simulink model "EV_thermal_charger_2015a_20200311"  (R2015a)
settings: Solver=ode3  StartTime=0.0  StopTime=1800  FixedStep=sampling_time  RelTol=1e-3
PreLoadFcn:
  | run('init_setting.m')
PostLoadFcn:
  | set_param(gcs, 'SimulationCommand', 'update');
  | load('save_param/save_P_Charger', 'P_Charger');
  | load('save_param/save_T_User_set_temp_degC','T_User_set_temp_degC');
  | load('save_param/save_ENV_PNT_PTTH_Temp_add_degC','ENV_PNT_PTTH_Temp_add_degC');
  | load('save_param/save_ENV_PNT_CABIN_Temp_add_degC','ENV_PNT_CABIN_Temp_add_degC');
  | load('save_param/save_ENV_PNT_PHI_Sunlight_W','ENV_PNT_PHI_Sunlight_W');
  | load('save_param/save_ENV_PNT_Outside_Temp_ini_degC','ENV_PNT_Outside_Temp_ini_degC');
undefined symbols (not defined in the file or in its folder): BK_PNT_Pow_UL, BK_PNT_ReGene_vel_limit_DN_kmph, BK_PNT_ReGene_vel_limit_UP_kmph, BK_PNT_Tau_brake, Brk_LL, Brk_PGain, Brk_UL, BT_PNT_Hi_C_pol_hi_batt, BT_PNT_Hi_Capa_hi_batt_F, BT_PNT_Hi_ocv_SOC_hi_batt_OCV_V_table, BT_PNT_Hi_ocv_SOC_hi_batt_OCV_V_table_x_SOC, BT_PNT_Hi_R_hi_batt_cell, BT_PNT_Hi_R_pol_hi_batt, BT_PNT_Hi_SOC_MAX_hi_batt, BT_PNT_Hi_SOC_MIN_hi_batt, BT_PNT_Hi_SOC_START_hi_batt, BT_PNT_Lo_Capa_lo_batt_F, BT_PNT_Lo_ocv_SOC_lo_batt_OCV_V_table, BT_PNT_Lo_ocv_SOC_lo_batt_OCV_V_table_x_SOC, BT_PNT_Lo_R_lo_batt_ohm, BT_PNT_Lo_SOC_MAX_lo_batt, BT_PNT_Lo_SOC_MIN_lo_batt, BT_PNT_Lo_SOC_START_lo_batt, BTTH_CNT_P_BT_Heater_W, BTTH_CNT_P_BT_Heater_W_x_BTCells_degC, BTTH_CNT_Voltage_BTFan_V, BTTH_CNT_Voltage_BTFan_V_x_BTCells_degC, BTTH_PNT_BT_Heat_Resi_KpW, BTTH_PNT_BT_Heat_Resi_KpW_x_Wind_m3ps, BTTH_PNT_BT_Heater2BTCells_Heat_Resi_KpW, BTTH_PNT_BT_Heater_Heat_Capa_JpK, BTTH_PNT_BTBlock2BTAir_Heat_Resi_KpW, BTTH_PNT_BTBlock_Heat_Capa_JpK, BTTH_PNT_BTCells2BTBlock_Heat_Resi_KpW, BTTH_PNT_BTCells_Heat_Capa_JpK, BTTH_PNT_v_BTFan_Wind_vel_mps, BTTH_PNT_v_BTFan_Wind_vel_mps_x_V_BTFan, CATH_CNT_P_Aircon_W_LL, CATH_CNT_P_Aircon_W_UL, CATH_CNT_P_Gain_Aircon, CATH_CNT_P_Gain_PTC_Heater, CATH_CNT_P_Gain_SeatHT, CATH_CNT_P_PTC_Heater, CATH_CNT_P_PTC_Heater_W_LL, CATH_CNT_P_PTC_Heater_W_UL, CATH_CNT_P_PTC_Heater_x_T_Outside_temp_degC, CATH_CNT_P_SeatHT_W_LL, CATH_CNT_P_SeatHT_W_UL, CATH_CNT_PGain_Temp_blowout, CATH_CNT_T_Aircon_Indoor_degC, CATH_CNT_T_Aircon_Indoor_degC_x_T_blowout_degC, CATH_CNT_T_PTC_Heater_degC_UL, CATH_CNT_T_SeatHT_Temp_degC, CATH_CNT_T_SeatHT_Temp_degC_x_T_blowout_degC, CATH_CNT_V_HVAC_Fan, CATH_CNT_V_HVAC_Fan_x_T_blowout_degC, CATH_CNT_V_RDFan_V, CATH_CNT_V_RDFan_x_P_Aircon_W, CATH_PNT_Air_Convection_Heat_Resi_KpW, CATH_PNT_Air_Convection_Heat_Resi_x_mps ... (+141)
undefined symbols (not defined in the file): ACC_D_Gain, ACC_I_Gain, ACC_P_Gain
libraries: METI_Lib_vehicle_model x52, simulink x35
(part 1 of 6)
PreSaveFcn:
  | save('save_param/save_P_Charger', 'P_Charger');
  | save('save_param/save_T_User_set_temp_degC', 'T_User_set_temp_degC');
  | save('save_param/save_ENV_PNT_PTTH_Temp_add_degC', 'ENV_PNT_PTTH_Temp_add_degC');
  | save('save_param/save_ENV_PNT_CABIN_Temp_add_degC', 'ENV_PNT_CABIN_Temp_add_degC');
  | save('save_param/save_ENV_PNT_PHI_Sunlight_W', 'ENV_PNT_PHI_Sunlight_W');
  | save('save_param/save_ENV_PNT_Outside_Temp_ini_degC', 'ENV_PNT_Outside_Temp_ini_degC');
settings Model: Creator=AZAPA  LastModifiedBy=itc-38
settings OptimizationCC: EfficientMapNaN2IntZero=off
settings DebuggingCC: SFInvalidInputDataAccessInChartInitDiag=none  SFNoUnconditionalDefaultTransitionDiag=none
settings HardwareCC: TargetLongLongMode=on  TargetIntDivRoundTo=Zero  TargetEndianess=LittleEndian  TargetHWDeviceType=MATLAB Host  ProdEqTarget=off
settings CodeAppCC: MaxIdLength=128
settings GRTTargetCC: CombineOutputUpdateFcns=off  GRTInterface=on

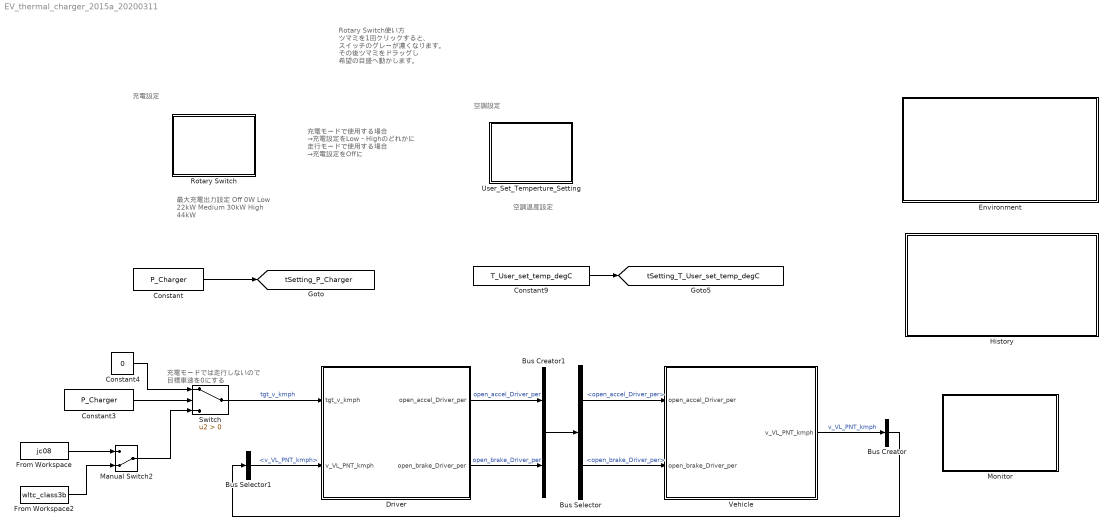
== system EV_thermal_charger_2015a_20200311 ==
  note: 充電モードでは走行しないので
      | 目標車速を0にする
  note: 充電モードで使用する場合
      | →充電設定をLow～Highのどれかに
      |
      | 走行モードで使用する場合
      | →充電設定をOffに
  note: 充電設定
  note: 空調温度設定
  note: 空調設定
  note: 最大充電出力設定
      | Off 0W
      | Low 22kW
      | Medium 30kW
      | High 44kW
  note: Rotary Switch使い方
      | ツマミを1回クリックすると、
      | スイッチのグレーが濃くなります。
      | その後ツマミをドラッグし
      | 希望の目盛へ動かします。
  Bus Creator : BusCreator  Inputs=1
  Bus Creator1 : BusCreator  Inputs=2
  Bus Selector : BusSelector  OutputSignals=open_accel_Driver_per,open_brake_Driver_per
  Bus Selector1 : BusSelector  OutputSignals=v_VL_PNT_kmph
  Constant : Constant  Value=P_Charger
  Constant3 : Constant  Value=P_Charger
  Constant4 : Constant  Value=0
  Constant9 : Constant  Value=T_User_set_temp_degC
  Driver : Subsystem
      mask Display: image(imread('picture\ドライバ.png'))
  Environment : Subsystem
  From Workspace : FromWorkspace  VariableName=jc08  SampleTime=0
  From Workspace2 : FromWorkspace  VariableName=wltc_class3b  SampleTime=0
  History : Subsystem
  Manual Switch2 : ManualSwitch  CurrentSetting=0
  Monitor : Subsystem
  Rotary Switch : Subsystem  DialogController=hmiCreateDDGDialog  IsWebBlock=on  mask(MathWorksWebBlock){webBlockId=86bdfb7e-e008-490f-bc47-d07dc2166084, webBlockType=discreteknob, ShowInLibBrowser=on, ShowInitialText=on, HMISrcModelName=EV_thermal_charger_2015a_20200311}
      mask prompts: webBlockId "WebBlock Id"; webBlockType "WebBlock Type"; HMISrcModelName "Source Model"
      mask Help: helpview([docroot '/mapfiles/simulink.map'], 'hmi_rotary_switch')
      mask Display:
      | model = bdroot(gcb);
      | if strcmp(get_param(model,'BlockDiagramType'), 'library')
      |     image([(matlabroot) '/toolbox/simulink/hmi/icons/DiscreteKnob.png']);
      | end
  Switch : Switch  Criteria=u2 > Threshold
  User_Set_Temperture_Setting : Subsystem  DialogController=hmiCreateDDGDialog  IsWebBlock=on  mask(MathWorksWebBlock){webBlockId=2ed6c567-8d1a-4bfe-bbc2-8860f67c8545, webBlockType=discreteknob, ShowInLibBrowser=on, ShowInitialText=on, HMISrcModelName=EV_thermal_charger_2015a_20200311}
      mask prompts: webBlockId "WebBlock Id"; webBlockType "WebBlock Type"; HMISrcModelName "Source Model"
      mask help: 値を設定してパラメーターまたは変数を調整します。
      mask Help: helpview([docroot '/mapfiles/simulink.map'], 'hmi_rotary_switch')
      mask Display:
      | if strcmp(get_param(bdroot(gcb),'BlockDiagramType'),'library')
      |  image([(matlabroot) '/toolbox/simulink/hmi/icons/DiscreteKnob.png'])
      | end
  Vehicle : Subsystem
      mask Display: image(imread('picture\電気負荷.png'))
  tag scope: tSetting_P_Charger=global, tSetting_T_User_set_temp_degC=global
  wires:
  Switch/1 -> Driver/1(tgt_v_kmph)  "tgt_v_kmph"
  From Workspace/1 -> Manual Switch2/1
  From Workspace2/1 -> Manual Switch2/2
  Vehicle/1(v_VL_PNT_kmph) -> Bus Creator/1  "v_VL_PNT_kmph"
  Bus Selector/1 -> Vehicle/1(open_accel_Driver_per)  "<open_accel_Driver_per>"
  Bus Selector/2 -> Vehicle/2(open_brake_Driver_per)  "<open_brake_Driver_per>"
  Bus Creator1/1 -> Bus Selector/1
  Driver/1(open_accel_Driver_per) -> Bus Creator1/1  "open_accel_Driver_per"
  Driver/2(open_brake_Driver_per) -> Bus Creator1/2  "open_brake_Driver_per"
  Bus Creator/1 -> Bus Selector1/1
  Bus Selector1/1 -> Driver/2(v_VL_PNT_kmph)  "<v_VL_PNT_kmph>"
  Manual Switch2/1 -> Switch/3
  Constant3/1 -> Switch/2
  Constant4/1 -> Switch/1
  Constant/1 -> [tSetting_P_Charger]
  Constant9/1 -> [tSetting_T_User_set_temp_degC]

== system EV_thermal_charger_2015a_20200311/Driver ==
  tgt_v_kmph : Inport
  v_VL_PNT_kmph : Inport  Port=2
  Caliculate_Driving_State : Subsystem
  Caliculate_Opeining_Accel : Subsystem
  Caliculate_Opening_Brake : Subsystem
  Memory2 : Memory  InheritSampleTime=on
  open_accel_Driver_per : Outport
  open_brake_Driver_per : Outport  Port=2
  tag scope: tScope_accel=global, tScope_brake=global, tScope_v_Vehicle=global, tScope_v_tgt=global
  wires:
  tgt_v_kmph/1 -> Caliculate_Driving_State/2(tgt_v_kmph), Caliculate_Opening_Brake/2(tgt_v_kmph), Caliculate_Opeining_Accel/2(tgt_v_kmph), [tScope_v_tgt]
  Memory2/1 -> [tScope_v_Vehicle], Caliculate_Opening_Brake/1(v_VL_PNT_kmph), Caliculate_Opeining_Accel/1(v_VL_PNT_kmph)
  Caliculate_Opeining_Accel/1(open_accel_Driver_per) -> open_accel_Driver_per/1, [tScope_accel], Caliculate_Opening_Brake/3(open_accel_Driver_per)
  Caliculate_Opening_Brake/1(open_brake_Driver_per) -> open_brake_Driver_per/1, [tScope_brake], Caliculate_Driving_State/1(open_brake_Driver_per)
  v_VL_PNT_kmph/1 -> Memory2/1

== system EV_thermal_charger_2015a_20200311/Environment ==
  note: 車外気温設定
      | VeryCold -30℃
      | Cold 0℃
      | Warm 20℃
      | VeryHot 40℃
  note: 気象設定（直射日光の有無）
      | Night 日射熱量 0W
      | Cloudy 日射熱量 100W
      | Sunny 日射熱量 1000W
  note: 気象条件設定
  note: Rotary Switch使い方
      | ツマミを1回クリックすると、
      | スイッチのグレーが濃くなります。
      | その後ツマミをドラッグし
      | 希望の目盛へ動かします。
  note: スタート時
      | 車室温度設定
      | 直射日光下で駐車した状態では
      | 車室温度は外気温より高くなる
  note: スタート時パワトレ・パワエレ
      | HOT/COLD設定
      | COLD 外気温と同じ温度から
      | HOT 外気温+40℃から
  note: 車両条件設定
  CABIN_Temp_add : Subsystem  DialogController=hmiCreateDDGDialog  IsWebBlock=on  mask(MathWorksWebBlock){webBlockId=d78e8cf1-5ca2-40c7-aa2c-f2b450f5124d, webBlockType=discreteknob, ShowInLibBrowser=on, ShowInitialText=on, HMISrcModelName=[]}
      mask prompts: webBlockId "WebBlock Id"; webBlockType "WebBlock Type"; HMISrcModelName "Source Model"
      mask help: 値を設定してパラメーターまたは変数を調整します。
      mask Help: helpview([docroot '/mapfiles/simulink.map'], 'hmi_rotary_switch')
      mask Display:
      | if strcmp(get_param(bdroot(gcb),'BlockDiagramType'),'library')
      |  image([(matlabroot) '/toolbox/simulink/hmi/icons/DiscreteKnob.png'])
      | end
  COLD/HOT : Subsystem  DialogController=hmiCreateDDGDialog  IsWebBlock=on  mask(MathWorksWebBlock){webBlockId=64b15bba-436a-47d2-9f2c-332ccf488184, webBlockType=discreteknob, ShowInLibBrowser=on, ShowInitialText=on, HMISrcModelName=[]}
      mask prompts: webBlockId "WebBlock Id"; webBlockType "WebBlock Type"; HMISrcModelName "Source Model"
      mask help: 値を設定してパラメーターまたは変数を調整します。
      mask Help: helpview([docroot '/mapfiles/simulink.map'], 'hmi_rotary_switch')
      mask Display:
      | if strcmp(get_param(bdroot(gcb),'BlockDiagramType'),'library')
      |  image([(matlabroot) '/toolbox/simulink/hmi/icons/DiscreteKnob.png'])
      | end
  Constant5 : Constant  Value=ENV_PNT_PTTH_Temp_add_degC
  Constant6 : Constant  Value=ENV_PNT_CABIN_Temp_add_degC
  Constant7 : Constant  Value=ENV_PNT_PHI_Sunlight_W
  Constant8 : Constant  Value=ENV_PNT_Outside_Temp_ini_degC
  Outside_Temperture_Setting : Subsystem  DialogController=hmiCreateDDGDialog  IsWebBlock=on  mask(MathWorksWebBlock){webBlockId=e3e71119-3dae-4264-804d-d3a93d53d578, webBlockType=discreteknob, ShowInLibBrowser=on, ShowInitialText=on, HMISrcModelName=[]}
      mask prompts: webBlockId "WebBlock Id"; webBlockType "WebBlock Type"; HMISrcModelName "Source Model"
      mask help: 値を設定してパラメーターまたは変数を調整します。
      mask Help: helpview([docroot '/mapfiles/simulink.map'], 'hmi_rotary_switch')
      mask Display:
      | if strcmp(get_param(bdroot(gcb),'BlockDiagramType'),'library')
      |  image([(matlabroot) '/toolbox/simulink/hmi/icons/DiscreteKnob.png'])
      | end
  Sunlight_Heat_Flux_Setting : Subsystem  DialogController=hmiCreateDDGDialog  IsWebBlock=on  mask(MathWorksWebBlock){webBlockId=802d8e5a-7805-4abc-9448-1c2511a8212f, webBlockType=discreteknob, ShowInLibBrowser=on, ShowInitialText=on, HMISrcModelName=[]}
      mask prompts: webBlockId "WebBlock Id"; webBlockType "WebBlock Type"; HMISrcModelName "Source Model"
      mask help: 値を設定してパラメーターまたは変数を調整します。
      mask Help: helpview([docroot '/mapfiles/simulink.map'], 'hmi_rotary_switch')
      mask Display:
      | if strcmp(get_param(bdroot(gcb),'BlockDiagramType'),'library')
      |  image([(matlabroot) '/toolbox/simulink/hmi/icons/DiscreteKnob.png'])
      | end
  tag scope: PHI_Environment_Sunlight_W=global, add_T_Environment_CATH_degC=global, add_T_Environment_PTTH_ELTH_degC=global, ini_T_Environment_Outside_degC=global
  wires:
  Constant7/1 -> [PHI_Environment_Sunlight_W]
  Constant8/1 -> [ini_T_Environment_Outside_degC]
  Constant5/1 -> [add_T_Environment_PTTH_ELTH_degC]
  Constant6/1 -> [add_T_Environment_CATH_degC]

== system EV_thermal_charger_2015a_20200311/History ==

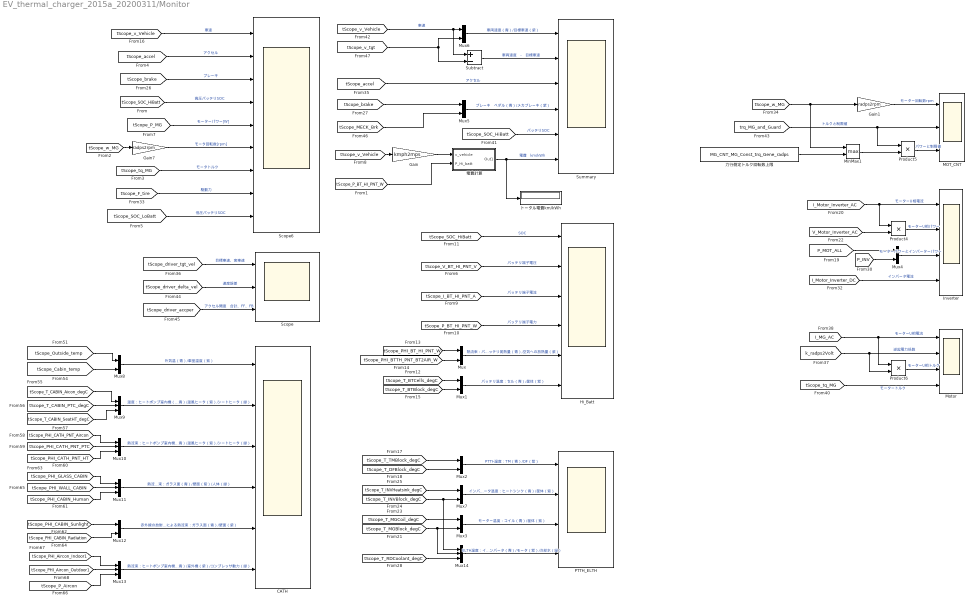
== system EV_thermal_charger_2015a_20200311/Monitor ==
  CATH : Scope  NumInputPorts=6
      settings: YMin=20~20~-35000~-0~0~-15000  YMax=70~70~5000~4500~1000~35000  SaveName=ScopeData12
  Gain : Gain  Gain=kmph2mps
  Gain1 : Gain  Gain=radps2rpm
  Gain7 : Gain  Gain=radps2rpm
  Hi_Batt : Scope  NumInputPorts=6
      settings: YMin=44.5~337.5~-100~-40000~-100~20  YMax=50~352.5~125~40000~1000~20.4  SaveName=ScopeData4
  Inverter : Scope  NumInputPorts=4
      settings: TimeRange=1800  YMin=-30~-7500~-12500~-30  YMax=60~15000~22500~60  SaveName=ScopeData15
  MOT_CNT : Scope  NumInputPorts=3
      settings: TimeRange=1800  YMin=-500~-350~-125000  YMax=7000~350~125000  SaveName=ScopeData11
  MinMax1 : MinMax  Function=max  Inputs=2
  Motor : Scope  NumInputPorts=4
      settings: TimeRange=1800  YMin=-2.5~0.75~-5~-10  YMax=35~1.025~40~100  SaveName=ScopeData14
  Mux{,1..8,12} (10 alike) : Mux  Inputs=2
  Mux{9..11,13..14} (5 alike) : Mux  Inputs=3
  PTTH_ELTH : Scope  NumInputPorts=4
      settings: TimeRange=1800  YMin=40~40~40~40  YMax=41~41.75~42~42  SaveName=ScopeData10
  Product4 : Product
  Product5 : Product
  Product6 : Product
  Scope : Scope  NumInputPorts=3
      settings: TimeRange=1800  YMin=0~-0.4~-20  YMax=140~1.2~80  SaveName=ScopeData8
  Scope6 : Scope  NumInputPorts=9
      settings: TimeRange=186.7025  YMin=35~0~-1~45.37~-30000~2250~-100~-3000~74.175  YMax=55~50~1~45.48~30000~4000~100~2000~74.35  SaveName=ScopeData6
  Subtract : Sum  Inputs=+-
  Summary : Scope  NumInputPorts=6
      settings: YMin=0~-0.6~0~0~41~0  YMax=150~0.1~70~5~50~9  SaveName=ScopeData5
  トータル電費km/kWh : Display
  力行側定トルク回転数上限 : Constant  Value=MG_CNT_MG_Const_trq_Gene_radps
  電費計算 : Subsystem
  wires:
  [tScope_v_Vehicle] -> Scope6/1  "車速"
  [tScope_accel] -> Scope6/2  "アクセル"
  [tScope_brake] -> Scope6/3  "ブレーキ"
  [tScope_SOC_HiBatt] -> Scope6/4  "高圧バッテリSOC"
  Gain7/1 -> Scope6/6  "モータ回転数[rpm]"
  [tScope_tq_MG] -> Scope6/7  "モータトルク"
  [tScope_F_tire] -> Scope6/8  "駆動力"
  Mux4/1 -> Inverter/3  "モーターパワーとインバーターパワー"
  [I_Motor_Inverter_AC] -> Product4/1, Inverter/1  "モーターU相電流"
  Product4/1 -> Inverter/2  "モーターU相パワー"
  [V_Motor_Inverter_AC] -> Product4/2
  [P_MOT_ALL] -> Mux4/1
  [P_INV] -> Mux4/2
  [I_Motor_Inverter_DC] -> Inverter/4  "インバータ電流"
  [trq_MG_and_Guard] -> Product5/1, MOT_CNT/2  "トルクと制限値"
  Product5/1 -> MOT_CNT/3  "パワーと制限値"
  力行側定トルク回転数上限/1 -> MinMax1/2
  MinMax1/1 -> Product5/2
  Gain1/1 -> MOT_CNT/1  "モーター回転数rpm"
  [tScope_w_MG] -> MinMax1/1, Gain1/1
  [I_MG_AC] -> Product6/1, Motor/1  "モーターU相電流"
  [k_radps2Volt] -> Product6/2, Motor/2  "逆起電力係数"
  Product6/1 -> Motor/3  "モーターU相トルク"
  [tScope_tq_MG] -> Motor/4  "モータートルク"
  Mux5/1 -> Summary/4  "ブレーキ　ペダル（青）/メカブレーキ（紫）"
  [tScope_MECK_Brk] -> Mux5/2
  [tScope_v_Vehicle] -> Subtract/1, Mux6/1  "車速"
  Mux6/1 -> Summary/1  "車両速度（青）/目標車速（紫）"
  Subtract/1 -> Summary/2  "車両速度　-　目標車速"
  [tScope_SOC_HiBatt] -> Summary/5  "バッテリSOC"
  [tScope_v_tgt] -> Mux6/2, Subtract/2
  [tScope_accel] -> Summary/3  "アクセル"
  [tScope_brake] -> Mux5/1
  [tScope_w_MG] -> Gain7/1
  [tScope_driver_tgt_vel] -> Scope/1  "目標車速、実車速"
  [tScope_driver_delta_vel] -> Scope/2  "速度誤差"
  [tScope_driver_accper] -> Scope/3  "アクセル開度　合計、FF、FB"
  電費計算/1(Out1) -> トータル電費km/kWh/1, Summary/6  "電費　km/kWh"
  [tScope_Outside_temp] -> Mux8/1
  [tScope_Cabin_temp] -> Mux8/2
  Mux8/1 -> CATH/1  "外気温（青）/車室温度（紫）"
  Mux9/1 -> CATH/2  "温度：ヒートポンプ室内機（青）/温風ヒータ（紫）/シートヒータ（緑）"
  [tScope_T_CABIN_Aicon_degC] -> Mux9/1
  [tScope_T_CABIN_PTC_degC] -> Mux9/2
  [tScope_T_CABIN_SeatHT_degC] -> Mux9/3
  Mux10/1 -> CATH/3  "熱流束：ヒートポンプ室内機（青）/温風ヒータ（紫）/シートヒータ（緑）"
  [tScope_PHI_CATH_PNT_Aircon] -> Mux10/1
  [tScope_PHI_CATH_PNT_PTC] -> Mux10/2
  [tScope_PHI_CATH_PNT_HT] -> Mux10/3
  Mux11/1 -> CATH/4  "熱流束：ガラス面（青）/壁面（紫）/人体（緑）"
  Mux12/1 -> CATH/5  "赤外線の放射による熱流束：ガラス面（青）/壁面（紫）"
  [tScope_PHI_CABIN_Sunlight] -> Mux12/1
  [tScope_PHI_CABIN_Radiation] -> Mux12/2
  [tScope_PHI_WALL_CABIN] -> Mux11/2
  [tScope_PHI_GLASS_CABIN] -> Mux11/1
  [tScope_PHI_CABIN_Human] -> Mux11/3
  Mux13/1 -> CATH/6  "熱流束：ヒートポンプ室内機（青）/室外機（紫）/コンプレッサ動力（緑）"
  [tScope_PHI_Aircon_Outdoor1] -> Mux13/2
  [tScope_PHI_Aircon_Indoor1] -> Mux13/1
  [tScope_P_Aircon] -> Mux13/3
  [tScope_v_Vehicle] -> Gain/1
  [tScope_P_BT_HI_PNT_W] -> 電費計算/2(P_Hi_batt)
  [tScope_SOC_LoBatt] -> Scope6/9  "低圧バッテリSOC"
  [tScope_P_MG] -> Scope6/5  "モーターパワー[W]"
  [tScope_SOC_HiBatt] -> Hi_Batt/1  "SOC"
  [tScope_V_BT_HI_PNT_V] -> Hi_Batt/2  "バッテリ端子電圧"
  [tScope_I_BT_HI_PNT_A] -> Hi_Batt/3  "バッテリ端子電流"
  Mux1/1 -> Hi_Batt/6  "バッテリ温度：セル（青）/筐体（紫）"
  Mux/1 -> Hi_Batt/5  "熱流束：バッテリ発熱量（青）/空気への放熱量（紫）"
  [tScope_P_BT_HI_PNT_W] -> Hi_Batt/4  "バッテリ端子電力"
  [tScope_PHI_BT_HI_PNT_W] -> Mux/1
  [tScope_PHI_BTTH_PNT_BT2AIR_W] -> Mux/2
  [tScope_T_BTCells_degC] -> Mux1/1
  [tScope_T_BTBlock_degC] -> Mux1/2
  Gain/1 -> 電費計算/1(v_vehicle)
  [tScope_T_DFBlock_degC] -> Mux2/2
  [tScope_T_TMBlock_degC] -> Mux2/1
  [tScope_T_MGCoil_degC] -> Mux3/1
  [tScope_T_MGBlock_degC] -> Mux14/2, Mux3/2
  [tScope_T_INVHeatsink_degC] -> Mux7/1
  [tScope_T_INVBlock_degC] -> Mux14/1, Mux7/2
  [tScope_T_RDCoolant_degC] -> Mux14/3
  Mux2/1 -> PTTH_ELTH/1  "PTTH温度：TM（青）/DF（紫）"
  Mux7/1 -> PTTH_ELTH/2  "インバータ温度：ヒートシンク（青）/筐体（紫）"
  Mux3/1 -> PTTH_ELTH/3  "モーター温度：コイル（青）/筐体（紫）"
  Mux14/1 -> PTTH_ELTH/4  "ELTH温度：インバータ（青）/モータ（紫）/冷却水（緑）"

== system EV_thermal_charger_2015a_20200311/Rotary Switch ==

== system EV_thermal_charger_2015a_20200311/User_Set_Temperture_Setting ==

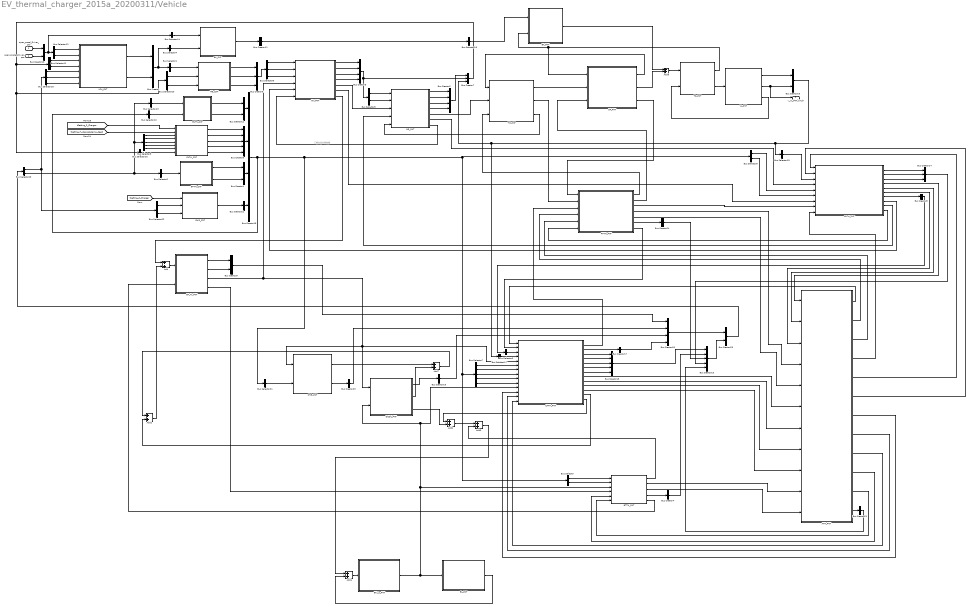
== system EV_thermal_charger_2015a_20200311/Vehicle ==
  note: 三相交流の実効値
  open_accel_Driver_per : Inport
  open_brake_Driver_per : Inport  Port=2
  ATM_PNT : Subsystem
  Add{,1..5,7} (7 alike) : Sum
  BK_CNT : Subsystem
      mask Display: image(imread('picture\ECU02.png'))
  BK_PNT : Subsystem
      mask Display: image(imread('picture\ブレーキ02.png'))
  BTTH_CNT : Subsystem
      mask Display: image(imread('ECU.png'))
  BTTH_PNT : Subsystem
      mask Display: image(imread('Li-INOバッテリ.png'))
  BT_Hi_PNT : Subsystem
      mask Display: image(imread('Li-INOバッテリ.png'))
  BT_Lo_PNT : Subsystem
      mask Display: image(imread('picture\バッテリー.png'))
  Bus Creator{,1,9..10,12,16,25} (7 alike) : BusCreator  Inputs=2
  Bus Creator{4,8,11,17,19,21..24} (9 alike) : BusCreator  Inputs=1
  Bus Creator13 : BusCreator  Inputs=5
  Bus Creator14 : BusCreator  Inputs=3
  Bus Creator15 : BusCreator  Inputs=5
  Bus Creator{2..3,18,20} (4 alike) : BusCreator
  Bus Creator5 : BusCreator  Inputs=5
  Bus Creator6 : BusCreator  Inputs=3
  Bus Creator7 : BusCreator  Inputs=3
  Bus Selector : BusSelector  OutputSignals=signal3.tgt_P_BTTH_CNT_BTHeater_W,signal3.V_BTTH_CNT_BTFan_V
  Bus Selector1 : BusSelector  OutputSignals=tgt_Trq_VCU_CNT_MG_Nm
  Bus Selector10 : BusSelector  OutputSignals=signal2.req_V_CATH_CNT_RDFan_V
  Bus Selector11 : BusSelector  OutputSignals=signal3.v_VL_PNT_mps_1,signal1.w_MG_PNT_radps
  Bus Selector12 : BusSelector  OutputSignals=open_brake_Driver_per,open_accel_Driver_per
  Bus Selector13 : BusSelector  OutputSignals=signal4.T_RDTH_PNT_RDCoolant_degC
  Bus Selector14 : BusSelector  OutputSignals=open_brake_Driver_per
  Bus Selector15 : BusSelector  OutputSignals=open_brake_BK_CNT_per
  Bus Selector16 : BusSelector  OutputSignals=signal3.v_VL_PNT_mps_1
  Bus Selector17 : BusSelector  OutputSignals=v_VL_PNT_kmps
  Bus Selector18 : BusSelector  OutputSignals=signal1.SOC_BT_Hi_PNT_per,signal4.P_HVAC_PNT_W,signal3.P_DCDC_PNT_W
  Bus Selector19 : BusSelector  OutputSignals=v_VL_PNT_kmps
  Bus Selector2 : BusSelector  OutputSignals=signal2.T_BC_PNT_degC
  Bus Selector20 : BusSelector  OutputSignals=signal1.w_MG_PNT_radps,signal2.V_INV_PNT_DC_V
  Bus Selector21 : BusSelector  OutputSignals=signal4.tgt_I_CHG_CNT_Charge_A
  Bus Selector22 : BusSelector  OutputSignals=signal2.V_CHG_PNT_V,signal1.SOC_BT_Hi_PNT_per
  Bus Selector23 : BusSelector  OutputSignals=signal1,signal2
  Bus Selector3 : BusSelector  OutputSignals=signal5.T_ATM_PNT_Outside_degC,signal1.T_CABA_PNT_degC,signal1.T_SH_PNT_degC,signal1.T_AC_PNT_Indoor_degC,signal1.T_PTC_PNT_degC
  Bus Selector4 : BusSelector  OutputSignals=F_VCU_CNT_re_break_N
  Bus Selector5 : BusSelector  OutputSignals=k_INV_PNT_Vpradps,Power_factor_INV_PNT
  Bus Selector6 : BusSelector  OutputSignals=Heat_Resi_ELTH_PNT_AirconCore_KpW
  Bus Selector7 : BusSelector  OutputSignals=signal2.P_CATH_CNT_Heatpomp_W,signal2.P_CATH_CNT_PTC_Heater_W,signal2.V_CATH_CNT_Aircon_Fan_V,signal2.P_CATH_CNT_SeatHT_W,signal1.req_V_ELTH_CNT_RDFan_V
  Bus Selector8 : BusSelector  OutputSignals=tgt_I_MG_CNT_UPhase_A,tgt_k_MG_CNT_Vpradps,Power_factor_MG_CNT
  Bus Selector9 : BusSelector  OutputSignals=signal1.req_V_ELTH_CNT_RDFan_V,signal1.V_ELTH_CNT_WP_V
  CATH_CNT : Subsystem
      mask Display: image(imread('ECU.png'))
  CATH_PNT : Subsystem
      mask Display: image(imread('熱マネ　カーエアコン.jpg'))
  CHG_CNT : Subsystem
      mask Display: image(imread('ECU.png'))
  CHG_PNT : Subsystem
      mask Display: image(imread('電気　有線充電器.jpg'))
  DCDC_PNT : Subsystem
      mask Display: image(imread('電気　降圧DCDCコンバータ.jpg'))
  DF_PNT : Subsystem
      mask Display: image(imread('picture\回転変換.png'))
  ELTH_CNT : Subsystem
      mask Display: image(imread('ECU.png'))
  ELTH_PNT : Subsystem
      mask Display: image(imread('picture\インバーター01.png'))
  EL_PNT : Subsystem
      mask Display: image(imread('picture\電気負荷.png'))
  INV_PNT : Subsystem
      mask Display: image(imread('picture\インバーター01.png'))
  MG_CNT : Subsystem
      mask Display: image(imread('picture\ECU03.png'))
  MG_PNT : Subsystem
      mask Display: image(imread('picture\モータドライブシステム03.png'))
  PTTH_PNT : Subsystem
      mask Display: image(imread('パワトレ　AT.jpg'))
  TM_PNT : Subsystem
      mask Display: image(imread('パワトレ　AT.jpg'))
  TR_PNT : Subsystem
      mask Display: image(imread('picture\タイヤ01.png'))
  VCU_CNT : Subsystem
      mask Display: image(imread('VCU.png'))
  VL_PNT : Subsystem
      mask Display: image(imread('自動車　EV車両.jpg'))
  v_VL_PNT_kmph : Outport
  wires:
  VCU_CNT/2(tgt_Trq_VCU_CNT_MG_Nm) -> Bus Creator/2  "tgt_Trq_VCU_CNT_MG_Nm"
  VCU_CNT/1(F_VCU_CNT_re_break_N) -> Bus Creator/1  "F_VCU_CNT_re_break_N"
  Bus Selector11/1 -> VCU_CNT/3(v_VL_PNT_mps_1)  "<v_VL_PNT_mps_1>"
  Bus Selector12/1 -> VCU_CNT/1(open_break_Driver_per)  "<open_brake_Driver_per>"
  Bus Selector12/2 -> VCU_CNT/2(open_accel_Driver_per)  "<open_accel_Driver_per>"
  Bus Selector11/2 -> VCU_CNT/4(w_MG_PNT_radps)  "<w_MG_PNT_radps>"
  Bus Selector18/1 -> VCU_CNT/5(SOC_BT_Hi_PNT_per)  "<SOC_BT_Hi_PNT_per>"
  open_brake_Driver_per/1 -> Bus Creator10/2
  open_accel_Driver_per/1 -> Bus Creator10/1
  TR_PNT/1(ｗ_TR_PNT_radps) -> DF_PNT/1("ｗ_TR_PNT_radps "), BK_PNT/2("w_TR_PNT_radps ")
  DF_PNT/2(Trq_DF_PNT_DN_Nm) -> Add5/2
  BT_Hi_PNT/3(V_BT_Hi_PNT_V) -> CATH_PNT/5(V_BT_Hi_PNT_V), CHG_PNT/1(V_BT_Hi_PNT_V), DCDC_PNT/1(V_BT_Hi_PNT_V), INV_PNT/4(V_BT_Hi_PNT_V)  "バッテリ電圧"
  BT_Lo_PNT/1("V_BT_Lo_PNT_V ") -> EL_PNT/1(V_BT_Lo_PNT_V), BTTH_PNT/3(V_BT_Lo_PNT_V), DCDC_PNT/2(V_BT_Lo_PNT_V), CATH_PNT/11(V_BT_Lo_PNT_V)
  BK_CNT/1(open_brake_BK_CNT_per) -> Bus Creator11/1  "open_brake_BK_CNT_per"
  MG_CNT/3(tgt_I_MG_CNT_UPhase_A) -> Bus Creator6/3  "tgt_I_MG_CNT_UPhase_A"
  MG_CNT/2(tgt_k_MG_CNT_Vpradps) -> Bus Creator6/2  "tgt_k_MG_CNT_Vpradps"
  INV_PNT/7(I_INV_PNT_DC_A) -> Add/1
  DCDC_PNT/2(I_DCDC_PNT_Hi_A) -> Add7/2
  Bus Selector1/1 -> MG_CNT/1(tgt_Trq_VCU_CNT_MG_Nm)  "<tgt_Trq_VCU_CNT_MG_Nm>"
  Bus Selector4/1 -> BK_CNT/2(F_VCU_CNT_re_brake_N)  "<F_VCU_CNT_re_break_N>"
  Bus Creator6/1 -> Bus Selector8/1
  Bus Selector20/1 -> MG_CNT/2(w_MG_PNT_radps)  "<w_MG_PNT_radps>"
  Bus Creator7/1 -> Bus Selector16/1, Bus Selector20/1, Bus Selector11/1
  Bus Creator16/1 -> Bus Creator7/3, Bus Selector17/1, Bus Selector19/1
  Bus Creator2/1 -> Bus Creator7/1
  Bus Selector20/2 -> MG_CNT/3(V_INV_PNT_DC_V)  "<V_INV_PNT_DC_V>"
  Bus Creator10/1 -> Bus Selector12/1, Bus Selector14/1
  Bus Selector14/1 -> BK_CNT/1(open_brake_Driver_per)  "<open_brake_Driver_per>"
  Bus Creator11/1 -> Bus Selector15/1
  Bus Selector15/1 -> BK_PNT/1(open_brake_BK_CNT_per)  "<open_brake_BK_CNT_per>"
  DCDC_PNT/1(P_DCDC_PNT_W) -> Bus Creator19/1  "P_DCDC_PNT_W"
  Bus Selector23/1 -> Bus Selector22/1, Bus Selector18/1  "<signal1>"
  TM_PNT/1("w_TM_PNT_DN_radps ") -> DF_PNT/2(w_TM_PNT_DN_radps)
  DF_PNT/1(Trq_DF_PNT_UP_Nm) -> TM_PNT/1(Trq_DF_PNT_UP_Nm)
  VL_PNT/1(v_VL_PNT_mps_1) -> Bus Creator16/1  "v_VL_PNT_mps_1"
  Add5/1 -> TR_PNT/1("Trq_TR_PNT_Nm ")
  BK_PNT/1(Trq_BK_PNT_Nm) -> Add5/1
  VL_PNT/3("v_VL_PNT_mps ") -> TR_PNT/2(v_VL_PNT_mps)
  TR_PNT/2("F_TR_PNT_N ") -> VL_PNT/1(F_TR_PNT_N)
  VL_PNT/2(v_VL_PNT_kmps) -> v_VL_PNT_kmph/1, Bus Creator16/2  "v_VL_PNT_kmps"
  BT_Hi_PNT/2(SOC_BT_Hi_PNT_per) -> Bus Creator9/2  "SOC_BT_Hi_PNT_per"
  BT_Hi_PNT/1(V_BT_Hi_PNT_V_1) -> Bus Creator9/1  "V_BT_Hi_PNT_V_1"
  Add/1 -> BT_Hi_PNT/1(I_BT_Hi_PNT_A)
  Add2/1 -> Add/2
  Bus Creator/1 -> Bus Selector1/1, Bus Selector4/1
  BT_Hi_PNT/4(PHI_BT_Hi_PNT_W) -> BTTH_PNT/4(PHI_BT_HI_PNT_W)
  BTTH_PNT/5(T_BC_PNT_K) -> BT_Hi_PNT/2(T_BC_PNT_K)
  ELTH_PNT/8(T_INVTH_PNT_K) -> INV_PNT/5(T_INVTH_PNT_K)
  INV_PNT/6(PHI_INV_PNT_W) -> ELTH_PNT/7(PHI_INV_PNT_W)
  MG_PNT/6("PHI_MG_PNT_W ") -> ELTH_PNT/4(PHI_MG_PNT_W)
  ELTH_PNT/9(T_MGTH_PNT_K) -> MG_PNT/4(T_MGTH_PNT_K)
  PTTH_PNT/2(T_DFTH_PNT_TM_K) -> DF_PNT/3("T_DFTH_PNT_TM_K ")
  DF_PNT/3("PHI_DF_PNT_W ") -> PTTH_PNT/1(PHI_DF_PNT_W)
  PTTH_PNT/1(T_TMTH_PNT_TM_K) -> TM_PNT/3(T_TMTH_PNT_TM_K)
  TM_PNT/2(PHI_TM_PNT_W) -> PTTH_PNT/2(PHI_TM_PNT_W)
  ATM_PNT/1(T_ATM_PNT_GL_K) -> CATH_PNT/1(T_ATM_PNT_GL_K)
  CATH_PNT/8(PHI_GL_PNT_ATM_W) -> ATM_PNT/6("PHI_GL_PNT_ATM_W ")
  ATM_PNT/8(T_ATM_PNT_WA_K) -> CATH_PNT/13(T_ATM_PNT_WA_K)
  CATH_PNT/9(PHI_WA_PNT_ATM_W) -> ATM_PNT/7("PHI_WA_PNT_ATM_W ")
  ATM_PNT/2(T_ATM_PNT_DF_K) -> PTTH_PNT/4(T_ATM_PNT_DF_K)
  PTTH_PNT/4("PHI_DFTH_PNT_ATM_W ") -> ATM_PNT/4(PHI_DFTH_PNT_ATM_W)
  ATM_PNT/3(T_ATM_PNT_TM_K) -> PTTH_PNT/5(T_ATM_PNT_TM_K)
  PTTH_PNT/5("PHI_TMTH_PNT_ATM_W ") -> ATM_PNT/5("PHI_TMTH_PNT_ATM_W ")
  ATM_PNT/5(T_ATM_PNT_RD_K) -> ELTH_PNT/1(T_ATM_PNT_RD_K)
  ELTH_PNT/5("PHI_RDTH_PNT_ATM_W ") -> ATM_PNT/2(PHI_RDTH_PNT_ATM_W)
  ATM_PNT/6(T_ATM_PNT_MG_K) -> ELTH_PNT/2(T_ATM_PNT_MG_K)
  ELTH_PNT/4("PHI_MGTH_PNT_ATM_W ") -> ATM_PNT/1(PHI_MGTH_PNT_ATM_W)
  ATM_PNT/4(T_ATM_PNT_INV_K) -> ELTH_PNT/9(T_ATM_PNT_INV_K)
  ELTH_PNT/6("PHI_INVTH_PNT_ATM_W ") -> ATM_PNT/3("PHI_INVTH_PNT_ATM_W ")
  ATM_PNT/10(T_ATM_PNT_BB_K) -> BTTH_PNT/5(T_ATM_PNT_BB_K)
  BTTH_PNT/2(PHI_BB_PNT_ATM_W) -> ATM_PNT/10(PHI_BB_PNT_ATM_W)
  ATM_PNT/11(T_ATM_PNT_BF_K) -> BTTH_PNT/6(T_ATM_PNT_BF_K)
  BTTH_PNT/3(PHI_BF_PNT_ATM_W) -> ATM_PNT/11(PHI_BF_PNT_ATM_W)
  PTTH_PNT/3(T_TMTH_PNT_ELTH_K) -> ELTH_PNT/8(T_TMTH_PNT_ELTH_K)
  ELTH_PNT/10(PHI_MGTH_PNT_PTTH_W) -> PTTH_PNT/6(PHI_MGTH_PNT_PTTH_W)
  BTTH_CNT/2(V_BTTH_CNT_BTFan_V) -> Bus Creator1/2  "V_BTTH_CNT_BTFan_V"
  BTTH_CNT/1(tgt_P_BTTH_CNT_BTHeater_W) -> Bus Creator1/1  "tgt_P_BTTH_CNT_BTHeater_W"
  Bus Selector/1 -> BTTH_PNT/1(tgt_P_BTTH_CNT_BTHeater_W)  "<tgt_P_BTTH_CNT_BTHeater_W>"
  Bus Selector/2 -> BTTH_PNT/2(V_BTTH_CNT_BTFan_V)  "<V_BTTH_CNT_BTFan_V>"
  BTTH_PNT/4(T_BC_PNT_degC) -> Bus Creator4/1  "T_BC_PNT_degC"
  Bus Selector2/1 -> BTTH_CNT/1(T_BC_PNT_degC)  "<T_BC_PNT_degC>"
  CATH_CNT/4(P_CATH_CNT_PTC_Heater_W) -> Bus Creator5/4  "P_CATH_CNT_PTC_Heater_W"
  CATH_CNT/3(req_V_CATH_CNT_RDFan_V) -> Bus Creator5/3  "req_V_CATH_CNT_RDFan_V"
  CATH_CNT/2(P_CATH_CNT_Heatpomp_W) -> Bus Creator5/2  "P_CATH_CNT_Heatpomp_W"
  CATH_CNT/1(V_CATH_CNT_Aircon_Fan_V) -> Bus Creator5/1  "V_CATH_CNT_Aircon_Fan_V"
  Bus Selector3/2 -> CATH_CNT/4(T_CABA_PNT_degC)  "<T_CABA_PNT_degC>"
  Bus Creator18/1 -> Bus Selector10/1, Bus Selector21/1, Bus Selector9/1, Bus Selector7/1, Bus Selector/1
  Bus Selector7/1 -> CATH_PNT/6(P_CATH_CNT_Heatpomp_W)  "<P_CATH_CNT_Heatpomp_W>"
  Bus Selector7/2 -> CATH_PNT/7(P_CATH_CNT_PTC_Heater_W)  "<P_CATH_CNT_PTC_Heater_W>"
  ELTH_CNT/1(req_V_ELTH_CNT_RDFan_V) -> Bus Creator12/1  "req_V_ELTH_CNT_RDFan_V"
  ELTH_CNT/2(V_ELTH_CNT_WP_V) -> Bus Creator12/2  "V_ELTH_CNT_WP_V"
  Bus Selector9/2 -> ELTH_PNT/6(V_ELTH_CNT_WP_V)  "<V_ELTH_CNT_WP_V>"
  Bus Selector9/1 -> ELTH_PNT/5(V_ELTH_CNT_RDFan_V)  "<req_V_ELTH_CNT_RDFan_V>"
  Bus Selector10/1 -> ELTH_CNT/2(req_V_CATH_CNT_RDFan_V)  "<req_V_CATH_CNT_RDFan_V>"
  ELTH_PNT/1(T_RDTH_PNT_RDCoolant_degC) -> Bus Creator14/1  "T_RDTH_PNT_RDCoolant_degC"
  Bus Selector13/1 -> ELTH_CNT/1(T_RDTH_PNT_RDCoolant_degC)  "<T_RDTH_PNT_RDCoolant_degC>"
  CATH_CNT/5(P_CATH_CNT_SeatHT_W) -> Bus Creator5/5  "P_CATH_CNT_SeatHT_W"
  Bus Selector19/1 -> ELTH_PNT/3(v_VL_PNT_kmph)  "<v_VL_PNT_kmps>"
  Bus Creator4/1 -> Bus Creator15/2
  Bus Creator14/1 -> Bus Creator15/4
  Bus Selector23/2 -> Bus Selector13/1, Bus Selector3/1, Bus Selector2/1  "<signal2>"
  Bus Creator1/1 -> Bus Creator18/3
  Bus Creator5/1 -> Bus Creator18/2
  Bus Creator12/1 -> Bus Creator18/1
  [tSetting_T_User_set_temp_degC] -> CATH_CNT/2(tSetting_T_User_set_temp_degC)
  Bus Selector3/1 -> CATH_CNT/3(T_ATM_PNT_Outside_degC)  "<T_ATM_PNT_Outside_degC>"
  CATH_PNT/11(T_GL_PNT_ATM_K) -> ATM_PNT/9(T_GL_PNT_ATM_K)
  ATM_PNT/7(PHI_ATM_PNT_Sunlight_W) -> CATH_PNT/12(PHI_ATM_PNT_Sunlight_W)
  Bus Creator19/1 -> Bus Creator20/3
  Bus Selector18/3 -> VCU_CNT/7(P_DCDC_PNT_W)  "<P_DCDC_PNT_W>"
  Bus Selector18/2 -> VCU_CNT/6(P_HVAC_PNT_W)  "<P_HVAC_PNT_W>"
  ATM_PNT/12(T_ATM_PNT_Outside_degC) -> Bus Creator21/1  "T_ATM_PNT_Outside_degC"
  Bus Creator21/1 -> Bus Creator15/5
  ELTH_PNT/2(T_MGTH_PNT_MGHousing_degC) -> Bus Creator14/2  "T_MGTH_PNT_MGHousing_degC"
  ELTH_PNT/3(T_INVTH_PNT_INVHeatsink_degC) -> Bus Creator14/3  "T_INVTH_PNT_INVHeatsink_degC"
  Bus Selector3/3 -> CATH_CNT/5(T_SH_PNT_degC)  "<T_SH_PNT_degC>"
  CHG_CNT/1(tgt_I_CHG_CNT_Charge_A) -> Bus Creator22/1  "tgt_I_CHG_CNT_Charge_A"
  Bus Selector21/1 -> CHG_PNT/2(tgt_I_CHG_CNT_Charge_A)  "<tgt_I_CHG_CNT_Charge_A>"
  CHG_PNT/2(V_CHG_PNT_V) -> Bus Creator23/1  "V_CHG_PNT_V"
  [tSetting_P_Charger] -> CHG_CNT/1(tSetting_P_Charger)
  PTTH_PNT/6(T_TMTH_PNT_TF_degC) -> Bus Creator24/1  "T_TMTH_PNT_TF_degC"
  Bus Creator24/1 -> Bus Creator15/3
  Bus Creator23/1 -> Bus Creator20/2
  Bus Selector22/1 -> CHG_CNT/2(V_CHG_PNT_V)  "<V_CHG_PNT_V>"
  Bus Selector22/2 -> CHG_CNT/3(SOC_BT_Hi_PNT_per)  "<SOC_BT_Hi_PNT_per>"
  Bus Creator22/1 -> Bus Creator18/4
  CATH_PNT/12(I_HVAC_PNT_A) -> Add2/2
  CHG_PNT/1(I_CHG_PNT_A) -> Add7/1
  Bus Selector7/3 -> CATH_PNT/8(V_CATH_CNT_Aircon_Fan_V)  "<V_CATH_CNT_Aircon_Fan_V>"
  Bus Selector7/4 -> CATH_PNT/9(P_CATH_CNT_SeatHT_W)  "<P_CATH_CNT_SeatHT_W>"
  DCDC_PNT/3(I_DCDC_PNT_Lo_A) -> Add1/2
  CATH_PNT/13(I_SH_PNT_A) -> Add1/1
  Add1/1 -> Add3/1
  BTTH_PNT/1(I_BTTH_PNT_A) -> Add3/2
  Add4/1 -> BT_Lo_PNT/1(I_BT_Lo_PNT_A)
  Add3/1 -> Add4/1
  EL_PNT/1(I_EL_PNT_A) -> Add4/2
  Add7/1 -> Add2/1
  CATH_PNT/3(T_AC_PNT_Outdoor_degC) -> Bus Creator13/1  "T_AC_PNT_Outdoor_degC"
  CATH_PNT/4(T_AC_PNT_Indoor_degC) -> Bus Creator13/2  "T_AC_PNT_Indoor_degC"
  CATH_PNT/5(T_PTC_PNT_degC) -> Bus Creator13/3  "T_PTC_PNT_degC"
  CATH_PNT/2(P_HVAC_PNT_W) -> Bus Creator17/1  "P_HVAC_PNT_W"
  Bus Creator17/1 -> Bus Creator20/4
  Bus Creator13/1 -> Bus Creator15/1
  Bus Selector3/4 -> CATH_CNT/6(T_AC_PNT_Indoor_degC)  "<T_AC_PNT_Indoor_degC>"
  Bus Selector3/5 -> CATH_CNT/7(T_PTC_PNT_degC)  "<T_PTC_PNT_degC>"
  Bus Selector16/1 -> CATH_CNT/8(v_vehicle_mps_1)  "<v_VL_PNT_mps_1>"
  ATM_PNT/9(T_ATM_PNT_AC_K) -> CATH_PNT/14(T_ATM_PNT_AC_K)
  CATH_PNT/10(PHI_AC_PNT_ATM_W) -> ATM_PNT/8(PHI_AC_PNT_ATM_W)
  Bus Selector7/5 -> CATH_PNT/10(req_V_ELTH_CNT_RDFan_V)  "<req_V_ELTH_CNT_RDFan_V>"
  Bus Selector17/1 -> CATH_PNT/4(v_VL_PNT_kmph)  "<v_VL_PNT_kmps>"
  CATH_PNT/6(T_CABA_PNT_degC) -> Bus Creator13/4  "T_CABA_PNT_degC"
  CATH_PNT/7(T_SH_PNT_degC) -> Bus Creator13/5  "T_SH_PNT_degC"
  ELTH_PNT/7(Heat_Resi_ELTH_PNT_AirconCore_KpW) -> Bus Creator8/1  "Heat_Resi_ELTH_PNT_AirconCore_KpW"
  Bus Creator8/1 -> Bus Selector6/1
  Bus Selector6/1 -> CATH_PNT/3(Heat_Resi_ELTH_PNT_AirconCore_KpW)  "<Heat_Resi_ELTH_PNT_AirconCore_KpW>"
  CATH_PNT/1(PHI_CATH_PNT_PTTH_W) -> PTTH_PNT/3("PHI_CATH_PNT_PTTH_W ")
  PTTH_PNT/7(T_PTTH_PNT_CATH_K) -> CATH_PNT/2(T_PTTH_PNT_CATH_K)
  [tSetting_P_Charger] -> CATH_CNT/1(tSetting_P_Charger)
  INV_PNT/1(k_INV_PNT_Vpradps) -> Bus Creator3/1  "k_INV_PNT_Vpradps"
  INV_PNT/5(I_INV_PNT_AC_A) -> MG_PNT/3("I_INV_PNT_AC_A ")
  MG_PNT/7("V_MG_PNT_AC_V ") -> INV_PNT/6(V_MG_PNT_AC_V)
  MG_PNT/1(w_MG_PNT_radps) -> Bus Creator2/1  "w_MG_PNT_radps"
  MG_PNT/2("Trq_MG_PNT_Nm_1 ") -> Bus Creator2/2  "Trq_MG_PNT_Nm_1"
  MG_PNT/3(V_MG_PNT_AC_V_1) -> Bus Creator2/3  "V_MG_PNT_AC_V_1"
  MG_PNT/4(I_MG_PNT_AC_A) -> Bus Creator2/4  "I_MG_PNT_AC_A"
  INV_PNT/3(V_INV_PNT_DC_V) -> Bus Creator3/3  "V_INV_PNT_DC_V"
  INV_PNT/4(I_INV_PNT_DC_A_1) -> Bus Creator3/4  "I_INV_PNT_DC_A_1"
  Bus Selector5/1 -> MG_PNT/1(k_MG_CNT_Vpradps)  "<k_INV_PNT_Vpradps>"
  Bus Selector8/1 -> INV_PNT/1(tgt_I_MG_CNT_UPhase_A)  "<tgt_I_MG_CNT_UPhase_A>"
  Bus Selector8/2 -> INV_PNT/2(tgt_k_MG_CNT_vpradps)  "<tgt_k_MG_CNT_Vpradps>"
  Bus Creator3/1 -> Bus Creator7/2, Bus Selector5/1
  TM_PNT/3(w_TM_PNT_UP_radps) -> MG_PNT/5(w_TM_PNT_UP_radps)
  MG_PNT/5(Trq_MG_PNT_Nm) -> TM_PNT/2("Trq_MG_PNT_Nm ")
  MG_CNT/1(Power_factor_MG_CNT) -> Bus Creator6/1  "Power_factor_MG_CNT"
  INV_PNT/2(Power_factor_INV_PNT) -> Bus Creator3/2  "Power_factor_INV_PNT"
  Bus Selector5/2 -> MG_PNT/2(Power_factor_INV_PNT)  "<Power_factor_INV_PNT>"
  Bus Selector8/3 -> INV_PNT/3(Power_factor_MG_CNT)  "<Power_factor_MG_CNT>"
  Bus Creator9/1 -> Bus Creator20/1
  Bus Creator20/1 -> Bus Creator25/1
  Bus Creator15/1 -> Bus Creator25/2
  Bus Creator25/1 -> Bus Selector23/1

== system EV_thermal_charger_2015a_20200311/Driver/Caliculate_Driving_State ==
  open_brake_Driver_per : Inport
  tgt_v_kmph : Inport  Port=2
  Constant : Constant  Value=Thresh_Stop_vCar
  Constant4 : Constant  Value=0.1*sampling_time
  Constant6 : Constant  Value=-0.1*sampling_time
  Memory : Memory
  Relational Operator : RelationalOperator  Operator=>  OutDataTypeStr=boolean
  Relational Operator1 : RelationalOperator  Operator=<  OutDataTypeStr=boolean
  Relational Operator2 : RelationalOperator  Operator=<  OutDataTypeStr=boolean
  Sum : Sum  Inputs=|+-
  Switch{,1..3} (4 alike) : Switch  Criteria=u2 > Threshold  Threshold=0.5
  Terminator : Terminator
  停止 : Constant  Value=drivmode_STOP
  加速 : Constant  Value=drivmode_ACC
  定常1 : Constant  Value=drivmode_CONST
  減速力行 : Constant  Value=drivmode_GensokuRikko
  減速回生 : Constant  Value=drivmode_GensokuKaisei
  wires:
  Switch/1 -> Terminator/1  "state_driving"
  tgt_v_kmph/1 -> Relational Operator/1, Memory/1, Sum/1
  Relational Operator1/1 -> Switch1/2
  Constant4/1 -> Relational Operator1/2
  Relational Operator/1 -> Switch/2
  Constant/1 -> Relational Operator/2
  停止/1 -> Switch/3
  Sum/1 -> Relational Operator1/1, Relational Operator2/1
  減速回生/1 -> Switch2/1
  Switch3/1 -> Switch1/1
  Constant6/1 -> Relational Operator2/2
  Memory/1 -> Sum/2
  open_brake_Driver_per/1 -> Switch2/2
  減速力行/1 -> Switch2/3
  Relational Operator2/1 -> Switch3/2
  Switch2/1 -> Switch3/1
  定常1/1 -> Switch3/3
  加速/1 -> Switch1/3
  Switch1/1 -> Switch/1

== system EV_thermal_charger_2015a_20200311/Driver/Caliculate_Opeining_Accel ==
  v_VL_PNT_kmph : Inport
  tgt_v_kmph : Inport  Port=2
  Constant : Constant  Value=VEHICLE_CNT_ACCper_UL
  Constant1 : Constant  Value=VEHICLE_CNT_ACCper_LL
  FB : Subsystem  mask{P_Gain=ACC_P_Gain, D_Gain=ACC_D_Gain, I_Gain=ACC_I_Gain}
      mask prompts: P_Gain "Pゲイン値"; D_Gain "Dゲイン値"; I_Gain "Iゲイン値"
  FF1 : Subsystem
  Mux : Mux  Inputs=2
  Mux1 : Mux  Inputs=3
  Saturation Dynamic : simulink/Discontinuities/Saturation Dynamic  OutMin=[]  OutMax=[]  OutDataTypeStr=Inherit: Same as second input  OutDataType=fixdt(1, 16)  OutScaling=2^-10  DoSatur=off
  Sum1 : Sum  Inputs=|-+
  Sum3 : Sum  Inputs=++|
  stopmode_calc : Subsystem
  open_accel_Driver_per : Outport
  tag scope: tScope_driver_accper=global, tScope_driver_delta_vel=global, tScope_driver_tgt_vel=global
  wires:
  Sum1/1 -> [tScope_driver_delta_vel], FB/1(delta_v_VL_kmph)
  v_VL_PNT_kmph/1 -> Mux/1, FF1/2(v_cal), Sum1/1
  Sum3/1 -> stopmode_calc/1(FF_FB_acc_per), Mux1/1
  FB/1(FB_open_accel_per) -> Sum3/1, Mux1/3
  FF1/1(per_acc_FF) -> Mux1/2, Sum3/2
  tgt_v_kmph/1 -> stopmode_calc/2(target_v_VL_kmph), FF1/1(v_tgt), Sum1/2, Mux/2
  Saturation Dynamic/1 -> open_accel_Driver_per/1  "open_accel_Driver_per"
  Mux/1 -> [tScope_driver_tgt_vel]  "目標車速 実車速"
  Mux1/1 -> [tScope_driver_accper]
  Constant/1 -> Saturation Dynamic/1
  Constant1/1 -> Saturation Dynamic/3
  stopmode_calc/1(open_accel_per) -> Saturation Dynamic/2

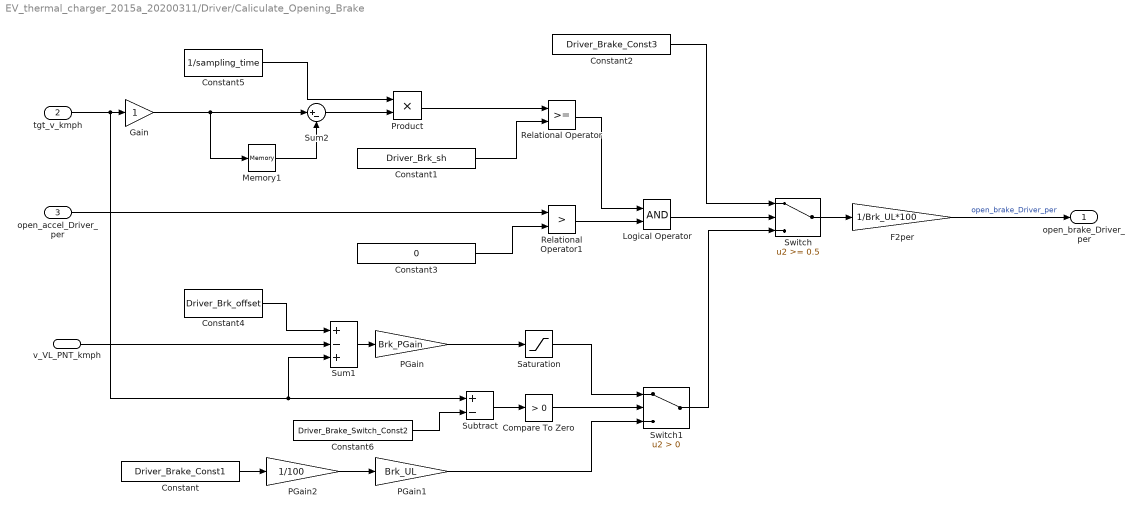
== system EV_thermal_charger_2015a_20200311/Driver/Caliculate_Opening_Brake ==
  v_VL_PNT_kmph : Inport
  tgt_v_kmph : Inport  Port=2
  open_accel_Driver_per : Inport  Port=3
  Compare To Zero : simulink/Logic and Bit Operations/Compare To Zero  relop=>  OutDataTypeStr=boolean
  Constant : Constant  Value=Driver_Brake_Const1
  Constant1 : Constant  Value=Driver_Brk_sh
  Constant2 : Constant  Value=Driver_Brake_Const3
  Constant3 : Constant  Value=0
  Constant4 : Constant  Value=Driver_Brk_offset
  Constant5 : Constant  Value=1/sampling_time
  Constant6 : Constant  Value=Driver_Brake_Switch_Const2
  F2per : Gain  Gain=1/Brk_UL*100
  Gain : Gain
  Logical Operator : Logic  AllPortsSameDT=off  OutDataTypeStr=boolean
  Memory1 : Memory
  PGain : Gain  Gain=Brk_PGain
  PGain1 : Gain  Gain=Brk_UL
  PGain2 : Gain  Gain=1/100
  Product : Product
  Relational Operator : RelationalOperator  OutDataTypeStr=boolean
  Relational Operator1 : RelationalOperator  Operator=>  OutDataTypeStr=boolean
  Saturation : Saturate  UpperLimit=Brk_UL  LowerLimit=Brk_LL
  Subtract : Sum  Inputs=+-
  Sum1 : Sum  Inputs=+-+
  Sum2 : Sum  Inputs=|+-
  Switch : Switch  Threshold=0.5
  Switch1 : Switch  Criteria=u2 > Threshold
  open_brake_Driver_per : Outport
  wires:
  tgt_v_kmph/1 -> Gain/1, Subtract/1, Sum1/3
  Sum1/1 -> PGain/1
  PGain/1 -> Saturation/1
  Constant/1 -> PGain2/1
  PGain1/1 -> Switch1/3
  open_accel_Driver_per/1 -> Relational Operator1/1
  Memory1/1 -> Sum2/2
  Switch/1 -> F2per/1
  Product/1 -> Relational Operator/1
  Saturation/1 -> Switch1/1
  Switch1/1 -> Switch/3
  Constant2/1 -> Switch/1
  Constant1/1 -> Relational Operator/2
  Constant3/1 -> Relational Operator1/2
  Relational Operator/1 -> Logical Operator/1
  Relational Operator1/1 -> Logical Operator/2
  F2per/1 -> open_brake_Driver_per/1  "open_brake_Driver_per"
  v_VL_PNT_kmph/1 -> Sum1/2
  Constant4/1 -> Sum1/1
  Sum2/1 -> Product/2
  Constant5/1 -> Product/1
  Constant6/1 -> Subtract/2
  Subtract/1 -> Compare To Zero/1
  Compare To Zero/1 -> Switch1/2
  Logical Operator/1 -> Switch/2
  PGain2/1 -> PGain1/1
  Gain/1 -> Memory1/1, Sum2/1

== system EV_thermal_charger_2015a_20200311/Environment/CABIN_Temp_add ==

== system EV_thermal_charger_2015a_20200311/Environment/COLD//HOT ==

== system EV_thermal_charger_2015a_20200311/Environment/Outside_Temperture_Setting ==

== system EV_thermal_charger_2015a_20200311/Environment/Sunlight_Heat_Flux_Setting ==

== system EV_thermal_charger_2015a_20200311/Monitor/電費計算 ==
  note: km
  note: m
  note: m/s
  note: W
  note: kWh
  note: kWsec
  note: Wsec
  v_vehicle : Inport
  P_Hi_batt : Inport  Port=2
  Constant : Constant  Value=0
  Divide_0wari : METI_Lib_vehicle_model/Divide_0wari
  Gain1 : Gain  Gain=1/1000
  Gain2 : Gain  Gain=1/3600
  Gain7 : Gain  Gain=1/1000
  Integrator : Integrator
  Integrator1 : Integrator
  Saturation Dynamic : simulink/Discontinuities/Saturation Dynamic  OutMin=[]  OutMax=[]  OutDataTypeStr=Inherit: Same as second input  OutDataType=fixdt(1, 16)  OutScaling=2^-10  DoSatur=off
  燃費表示上の上限値 : Constant  Value=50
  Out1 : Outport
  wires:
  Gain7/1 -> Divide_0wari/1
  燃費表示上の上限値/1 -> Saturation Dynamic/1
  Saturation Dynamic/1 -> Out1/1
  Divide_0wari/1 -> Saturation Dynamic/2
  Constant/1 -> Saturation Dynamic/3
  v_vehicle/1 -> Integrator/1
  Integrator/1 -> Gain7/1
  Gain2/1 -> Divide_0wari/2
  P_Hi_batt/1 -> Integrator1/1
  Integrator1/1 -> Gain1/1
  Gain1/1 -> Gain2/1

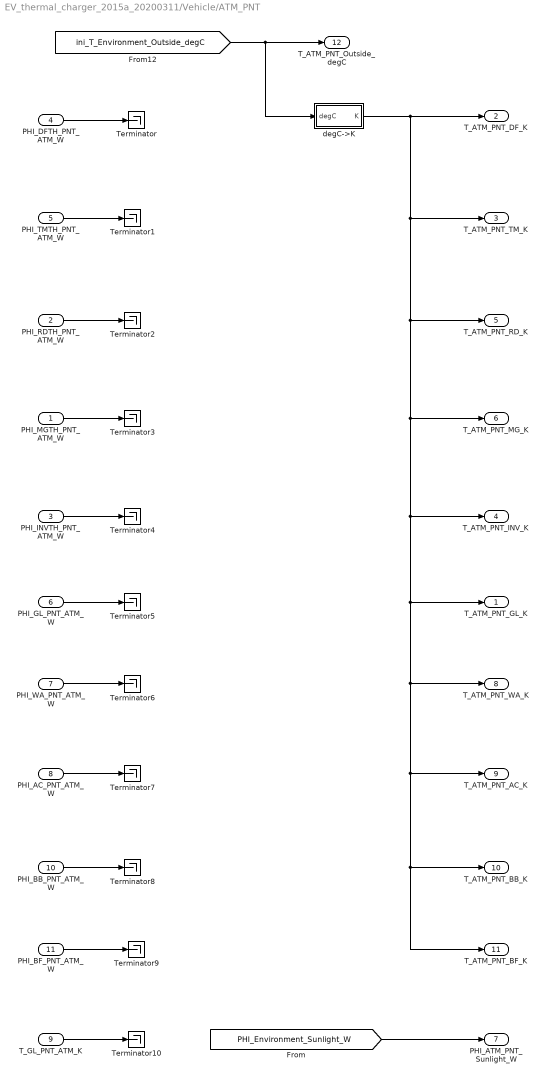
== system EV_thermal_charger_2015a_20200311/Vehicle/ATM_PNT ==
  PHI_MGTH_PNT_ATM_W : Inport
  PHI_RDTH_PNT_ATM_W : Inport  Port=2
  "PHI_INVTH_PNT_ATM_W " : Inport  Port=3
  PHI_DFTH_PNT_ATM_W : Inport  Port=4
  "PHI_TMTH_PNT_ATM_W " : Inport  Port=5
  "PHI_GL_PNT_ATM_W " : Inport  Port=6
  "PHI_WA_PNT_ATM_W " : Inport  Port=7
  PHI_AC_PNT_ATM_W : Inport  Port=8
  T_GL_PNT_ATM_K : Inport  Port=9
  PHI_BB_PNT_ATM_W : Inport  Port=10
  PHI_BF_PNT_ATM_W : Inport  Port=11
  Terminator{,1..10} (11 alike) : Terminator
  degC->K : Subsystem
  T_ATM_PNT_GL_K : Outport
  T_ATM_PNT_DF_K : Outport  Port=2
  T_ATM_PNT_TM_K : Outport  Port=3
  T_ATM_PNT_INV_K : Outport  Port=4
  T_ATM_PNT_RD_K : Outport  Port=5
  T_ATM_PNT_MG_K : Outport  Port=6
  PHI_ATM_PNT_Sunlight_W : Outport  Port=7
  T_ATM_PNT_WA_K : Outport  Port=8
  T_ATM_PNT_AC_K : Outport  Port=9
  T_ATM_PNT_BB_K : Outport  Port=10
  T_ATM_PNT_BF_K : Outport  Port=11
  T_ATM_PNT_Outside_degC : Outport  Port=12
  wires:
  [ini_T_Environment_Outside_degC] -> degC->K/1(degC), T_ATM_PNT_Outside_degC/1
  PHI_DFTH_PNT_ATM_W/1 -> Terminator/1
  "PHI_TMTH_PNT_ATM_W "/1 -> Terminator1/1
  PHI_RDTH_PNT_ATM_W/1 -> Terminator2/1
  PHI_MGTH_PNT_ATM_W/1 -> Terminator3/1
  "PHI_INVTH_PNT_ATM_W "/1 -> Terminator4/1
  "PHI_GL_PNT_ATM_W "/1 -> Terminator5/1
  "PHI_WA_PNT_ATM_W "/1 -> Terminator6/1
  PHI_AC_PNT_ATM_W/1 -> Terminator7/1
  PHI_BB_PNT_ATM_W/1 -> Terminator8/1
  PHI_BF_PNT_ATM_W/1 -> Terminator9/1
  degC->K/1(K) -> T_ATM_PNT_DF_K/1, T_ATM_PNT_TM_K/1, T_ATM_PNT_RD_K/1, T_ATM_PNT_MG_K/1, T_ATM_PNT_INV_K/1, T_ATM_PNT_GL_K/1, T_ATM_PNT_WA_K/1, T_ATM_PNT_AC_K/1, T_ATM_PNT_BF_K/1, T_ATM_PNT_BB_K/1
  [PHI_Environment_Sunlight_W] -> PHI_ATM_PNT_Sunlight_W/1
  T_GL_PNT_ATM_K/1 -> Terminator10/1

== system EV_thermal_charger_2015a_20200311/Vehicle/BK_CNT ==
  note: ～回生協調ブレーキ時～
      | 実際に出力できている回生ブレーキ力を受け取り
      | メカブレーキ負担分から減算することで
      | 車両としてのブレーキ力が
      | ドライバ操作通りになるようにする
  open_brake_Driver_per : Inport
  F_VCU_CNT_re_brake_N : Inport  Port=2
  Add : Sum
  Constant : Constant  Value=0
  Constant1 : Constant  Value=-inf
  Constant2 : Constant  Value=BK_PNT_Pow_UL
  Constant3 : Constant  Value=0
  Constant4 : Constant  Value=inf
  Constant5 : Constant  Value=BK_PNT_Pow_UL
  Divide : Product  Inputs=*/
  Product1 : Product
  Saturation Dynamic : simulink/Discontinuities/Saturation Dynamic  OutMin=[]  OutMax=[]  OutDataTypeStr=Inherit: Same as second input  OutDataType=fixdt(1, 16)  OutScaling=2^-10  DoSatur=off
  Saturation Dynamic1 : simulink/Discontinuities/Saturation Dynamic  OutMin=[]  OutMax=[]  OutDataTypeStr=Inherit: Same as second input  OutDataType=fixdt(1, 16)  OutScaling=2^-10  DoSatur=off
  per2F : Gain  Gain=1/100
  per2F1 : Gain  Gain=100
  open_brake_BK_CNT_per : Outport
  wires:
  F_VCU_CNT_re_brake_N/1 -> Saturation Dynamic/2  "F_VCU_CNT_re_brake_N"
  open_brake_Driver_per/1 -> per2F/1  "open_brake_Driver_per"
  Add/1 -> Saturation Dynamic1/2
  per2F/1 -> Product1/1
  Constant2/1 -> Product1/2
  Saturation Dynamic1/1 -> Divide/1
  Constant/1 -> Saturation Dynamic/1
  Constant1/1 -> Saturation Dynamic/3
  Constant3/1 -> Saturation Dynamic1/3
  Constant4/1 -> Saturation Dynamic1/1
  Product1/1 -> Add/1
  Saturation Dynamic/1 -> Add/2
  Constant5/1 -> Divide/2
  Divide/1 -> per2F1/1
  per2F1/1 -> open_brake_BK_CNT_per/1

== system EV_thermal_charger_2015a_20200311/Vehicle/BK_PNT ==
  note: 制動力
  open_brake_BK_CNT_per : Inport
  "w_TR_PNT_radps " : Inport  Port=2
  Constant2 : Constant  Value=tire_r
  Gain : Gain  Gain=-1
  Product6 : Product  RndMeth=Zero
  Q_cal3 : METI_Lib_vehicle_model/P_cal  Type_energy=回転運動  Type_output_energy=損失  Power_name=Pl_  t_Workspace_Name=BK_PNT_MECK_LOSS  P_VariableName=Pl_BK_PNT_MECK_LOSS  Across_VariableName=w_BK_PNT_MECK_LOSS  Throgh_VariableName=tq_BK_PNT_MECK_LOSS
  Terminator1 : Terminator
  Transfer Fcn : TransferFcn  Denominator=[BK_PNT_Tau_brake 1]
  per2F : Gain  Gain=BK_PNT_Pow_UL/100
  Trq_BK_PNT_Nm : Outport
  tag scope: tScope_MECK_Brk=global
  wires:
  Q_cal3/1 -> Terminator1/1
  Transfer Fcn/1 -> Product6/2
  Constant2/1 -> Product6/1
  Product6/1 -> Gain/1, Q_cal3/2
  "w_TR_PNT_radps "/1 -> Q_cal3/1
  open_brake_BK_CNT_per/1 -> [tScope_MECK_Brk], per2F/1
  Gain/1 -> Trq_BK_PNT_Nm/1  "trq_BK_PNT_Nm"
  per2F/1 -> Transfer Fcn/1

== system EV_thermal_charger_2015a_20200311/Vehicle/BTTH_CNT ==
  T_BC_PNT_degC : Inport
  1-D Lookup Table : Lookup_n-D  NumberOfTableDimensions=1  BreakpointsForDimension1=BTTH_CNT_P_BT_Heater_W_x_BTCells_degC  Table=BTTH_CNT_P_BT_Heater_W  InternalRulePriority=Speed  RndMeth=Simplest  InputSameDT=on
  1-D Lookup Table1 : Lookup_n-D  NumberOfTableDimensions=1  BreakpointsForDimension1=BTTH_CNT_Voltage_BTFan_V_x_BTCells_degC  Table=BTTH_CNT_Voltage_BTFan_V  InternalRulePriority=Speed  RndMeth=Simplest  InputSameDT=on
  tgt_P_BTTH_CNT_BTHeater_W : Outport
  V_BTTH_CNT_BTFan_V : Outport  Port=2
  wires:
  1-D Lookup Table/1 -> tgt_P_BTTH_CNT_BTHeater_W/1  "tgt_P_BTTH_CNT_BTHeater_W"
  1-D Lookup Table1/1 -> V_BTTH_CNT_BTFan_V/1  "V_BTTH_CNT_BTFan_V"
  T_BC_PNT_degC/1 -> 1-D Lookup Table1/1, 1-D Lookup Table/1  "T_BC_PNT_degC"

== system EV_thermal_charger_2015a_20200311/Vehicle/BTTH_PNT ==
  tgt_P_BTTH_CNT_BTHeater_W : Inport
  V_BTTH_CNT_BTFan_V : Inport  Port=2
  V_BT_Lo_PNT_V : Inport  Port=3
  PHI_BT_HI_PNT_W : Inport  Port=4
  T_ATM_PNT_BB_K : Inport  Port=5
  T_ATM_PNT_BF_K : Inport  Port=6
  BB_PNT : Subsystem
  BC_PNT : Subsystem
  BF_PNT : Subsystem
  BH_PNT : Subsystem
  K->degC : Subsystem
  K->degC1 : Subsystem
  I_BTTH_PNT_A : Outport
  PHI_BB_PNT_ATM_W : Outport  Port=2
  PHI_BF_PNT_ATM_W : Outport  Port=3
  T_BC_PNT_degC : Outport  Port=4
  T_BC_PNT_K : Outport  Port=5
  tag scope: tScope_PHI_BTTH_PNT_BT2AIR_W=global, tScope_T_BTBlock_degC=global, tScope_T_BTCells_degC=global
  wires:
  K->degC/1(degC) -> [tScope_T_BTCells_degC], T_BC_PNT_degC/1  "T_BTCells_degC"
  K->degC1/1(degC) -> [tScope_T_BTBlock_degC]
  [ini_T_Environment_Outside_degC] -> BH_PNT/1(ini_T_Environment_Outside_degC), BC_PNT/3(ini_T_Environment_Outside_degC), BB_PNT/1(ini_T_Environment_Outside_degC)
  tgt_P_BTTH_CNT_BTHeater_W/1 -> BH_PNT/2(tgt_P_BTTH_CNT_BTHeater_W)  "tgt_P_BTTH_CNT_BTHeater_W"
  V_BT_Lo_PNT_V/1 -> BH_PNT/3(V_BT_Lo_PNT_V)
  BH_PNT/2(I_BTTH_PNT_A) -> I_BTTH_PNT_A/1
  PHI_BT_HI_PNT_W/1 -> BC_PNT/5(PHI_BT_HI_PNT_W)
  BH_PNT/1(PHI_BTCells_Resi1_W) -> BC_PNT/4(PHI_BTCells2_W)
  BC_PNT/3(T_BC_PNT_K) -> T_BC_PNT_K/1
  BC_PNT/5(T_BTCells2_K) -> BH_PNT/4(T_BTCells_Resi1_K)
  BC_PNT/4(T_BTCCell_K) -> K->degC/1(K)
  V_BTTH_CNT_BTFan_V/1 -> BF_PNT/1(V_BTTH_CNT_BTFan_V)  "V_BTTH_CNT_BTFan_V"
  BC_PNT/1(T_BTCells4_K) -> BF_PNT/3(T_BT_Fan_Resi2_K)
  T_ATM_PNT_BF_K/1 -> BF_PNT/2(T_ATM_PNT_BF_K)
  BF_PNT/1(PHI_BT_Fan_Resi2_W) -> BC_PNT/1(PHI_BTCells4_W)
  BF_PNT/2(PHI_BF_PNT_ATM_W) -> PHI_BF_PNT_ATM_W/1
  BB_PNT/2(PHI_BB_PNT_ATM_W) -> PHI_BB_PNT_ATM_W/1, [tScope_PHI_BTTH_PNT_BT2AIR_W]
  BC_PNT/2(PHI_BTBlock_Resi1_W) -> BB_PNT/3(PHI_BTBlock1_W)
  T_ATM_PNT_BB_K/1 -> BB_PNT/2(T_ATM_PNT_BB_K)
  BB_PNT/1(T_BTBlock1_K) -> BC_PNT/2(T_BTBlock_Resi1_K)
  BB_PNT/3(T_BTBlock2_K) -> K->degC1/1(K)

== system EV_thermal_charger_2015a_20200311/Vehicle/BT_Hi_PNT ==
  note: SOC算出
  note: 内部抵抗
  note: OCV電圧算出
  I_BT_Hi_PNT_A : Inport
  T_BC_PNT_K : Inport  Port=2
  Cal_SOC : Subsystem
  Capa_batt(Ah) : Constant  Value=BT_PNT_Hi_Capa_hi_batt_F
  Gain : Gain  Gain=-1
  Memory6 : Memory  InheritSampleTime=on
  P_cal : METI_Lib_vehicle_model/P_cal  Type_energy=電気  Type_output_energy=出力  Power_name=Po_  t_Workspace_Name=BT_HI_PNT_ELEC  P_VariableName=Po_BT_HI_PNT_ELEC  Across_VariableName=V_BT_HI_PNT_ELEC  Throgh_VariableName=I_BT_HI_PNT_ELEC
  P_cal1 : METI_Lib_vehicle_model/P_cal  Type_energy=電気  Type_output_energy=損失  Power_name=Pl_  t_Workspace_Name=BT_PNT_HI_ELEC_LOSS  P_VariableName=Pl_BT_PNT_HI_ELEC_LOSS  Across_VariableName=V_BT_PNT_HI_ELEC_LOSS  Throgh_VariableName=I_BT_PNT_HI_ELEC_LOSS
  Product : Product
  SOC_MAX(%) : Constant  Value=BT_PNT_Hi_SOC_MAX_hi_batt
  SOC_MIN(%) : Constant  Value=BT_PNT_Hi_SOC_MIN_hi_batt
  SOC_START(%) : Constant  Value=BT_PNT_Hi_SOC_START_hi_batt
  Subsystem : Subsystem
  Sum : Sum
  Terminator1 : Terminator
  Terminator2 : Terminator
  map_OCV : Lookup  InputValues=BT_PNT_Hi_ocv_SOC_hi_batt_OCV_V_table_x_SOC  Table=BT_PNT_Hi_ocv_SOC_hi_batt_OCV_V_table  LookUpMeth=Interpolation-Use End Values
  V_BT_Hi_PNT_V_1 : Outport
  SOC_BT_Hi_PNT_per : Outport  Port=2
  V_BT_Hi_PNT_V : Outport  Port=3
  PHI_BT_Hi_PNT_W : Outport  Port=4
  tag scope: tScope_I_BT_HI_PNT_A=global, tScope_PHI_BT_HI_PNT_W=global, tScope_P_BT_HI_PNT_W=global, tScope_SOC_HiBatt=global, tScope_V_BT_HI_PNT_V=global
  wires:
  Capa_batt(Ah)/1 -> Cal_SOC/2(Capa_batt)
  SOC_START(%)/1 -> Cal_SOC/3(SOC_st)
  SOC_MAX(%)/1 -> Cal_SOC/4(SOC_MAX)
  SOC_MIN(%)/1 -> Cal_SOC/5(SOC_MIN)
  Sum/1 -> V_BT_Hi_PNT_V_1/1, Product/1, V_BT_Hi_PNT_V/1, [tScope_V_BT_HI_PNT_V], P_cal/1  "volt_BT_HI_PNT_V"
  map_OCV/1 -> Sum/1
  Subsystem/1(V_BT_PNT_V) -> P_cal1/1, Sum/2
  P_cal/1 -> Terminator2/1
  P_cal1/1 -> PHI_BT_Hi_PNT_W/1, [tScope_PHI_BT_HI_PNT_W]
  I_BT_Hi_PNT_A/1 -> Gain/1, Memory6/1
  Cal_SOC/1(SOC_out) -> SOC_BT_Hi_PNT_per/1, [tScope_SOC_HiBatt], map_OCV/1  "SOC_BT_HI_PNT_PCT"
  Memory6/1 -> Subsystem/1(I_BT_PNT_A), P_cal1/2, Cal_SOC/1(I_BT_PNT_A)
  T_BC_PNT_K/1 -> Terminator1/1
  Product/1 -> [tScope_P_BT_HI_PNT_W]
  Gain/1 -> [tScope_I_BT_HI_PNT_A], P_cal/2, Product/2
